simulink model "motor_speed"  (R2021b)
settings: Solver=FixedStepAuto  StartTime=0.0  StopTime=20  FixedStep=0.01  RelTol=1e-3
PreLoadFcn:
  | J = 0.01;
  | b = 0.1;
  | K = 0.01;
  | R = 1;
  | L = 0.5;
  | Ts = 0.01;
  | Kp = 210;
  | Ki = 630;
  | Kd = 20;
settings Model: Creator=adish  LastModifiedBy=adish
settings OptimizationCC: UseDivisionForNetSlopeComputation=on

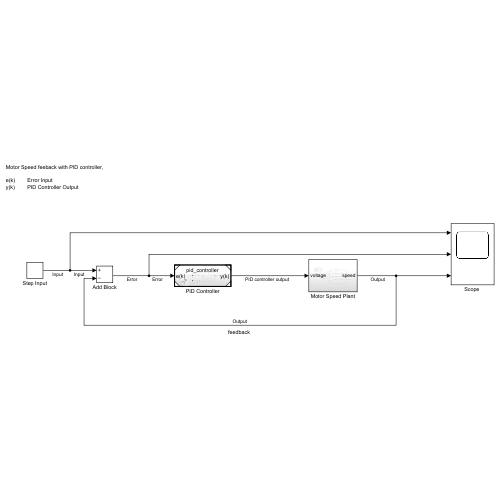
[thumbnail: Simulink's stored preview of the top-level diagram]
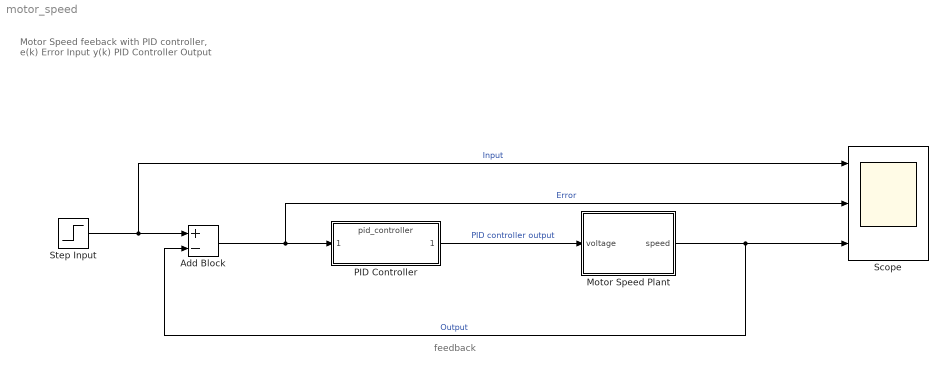
== system motor_speed ==
  note: Motor Speed feeback with PID controller,
      |
      | e(k)		Error Input
      | y(k)		PID Controller Output
  note: feedback
  Add Block : Sum  Inputs=+-
  Motor Speed Plant : Subsystem
  PID Controller : ModelReference  ModelNameDialog=pid_controller.slx  SimulationMode=Normal  ModelReferenceVersion=1.85
  "Scope " : Scope  NumInputPorts=3
  Step Input : Step  After=100  SampleTime=0
  wires:
  Step Input/1 -> "Scope "/1, Add Block/1  "Input"
  Add Block/1 -> "Scope "/2, PID Controller/1  "Error"
  PID Controller/1 -> Motor Speed Plant/1(voltage)  "PID controller output"
  Motor Speed Plant/1(speed) -> Add Block/2, "Scope "/3  "Output"

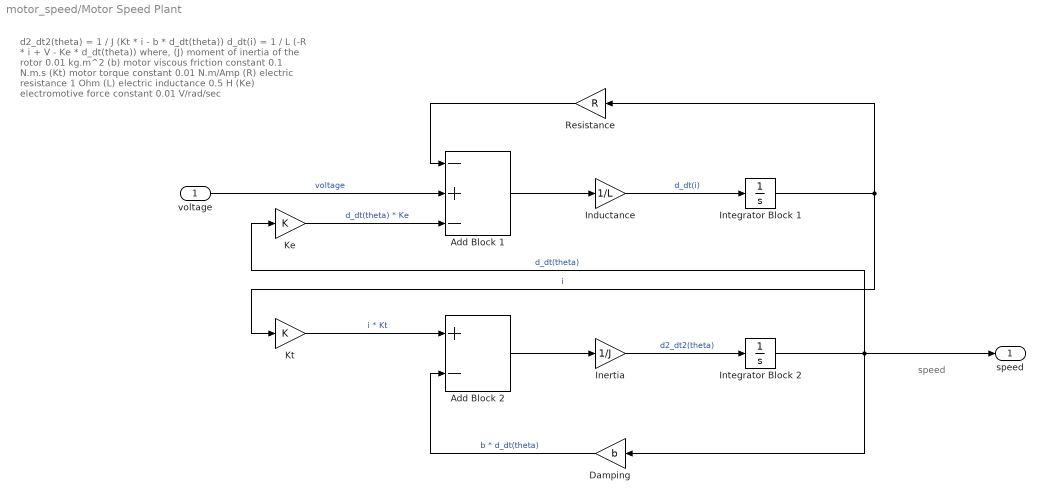
== system motor_speed/Motor Speed Plant ==
  note: speed
  note: d2_dt2(theta) = 1 / J (Kt * i - b * d_dt(theta))
      | d_dt(i) = 1 / L (-R * i + V - Ke * d_dt(theta))
      |
      | where,
      | (J) moment of inertia of the rotor 0.01 kg.m^2
      | (b) motor viscous friction constant 0.1 N.m.s
      | (Kt) motor torque constant 0.01 N.m/Amp
      | (R) electric resistance 1 Ohm
      | (L) electric inductance 0.5 H
      | (Ke) electromotive force constant 0.01 V/rad/sec
  voltage : Inport
  Add Block 1 : Sum  Inputs=-+-
  Add Block 2 : Sum  Inputs=+-
  Damping : Gain  Gain=b
  Inductance : Gain  Gain=1/L
  Inertia : Gain  Gain=1/J
  Integrator Block 1 : Integrator
  Integrator Block 2 : Integrator
  Ke : Gain  Gain=K
  Kt : Gain  Gain=K
  Resistance : Gain  Gain=R
  speed : Outport
  wires:
  Integrator Block 1/1 -> Kt/1, Resistance/1  "i"
  Add Block 2/1 -> Inertia/1
  Inertia/1 -> Integrator Block 2/1  "d2_dt2(theta)"
  Resistance/1 -> Add Block 1/1
  Add Block 1/1 -> Inductance/1
  Ke/1 -> Add Block 1/3  "d_dt(theta) * Ke"
  Damping/1 -> Add Block 2/2  "b * d_dt(theta)"
  Integrator Block 2/1 -> Damping/1, speed/1, Ke/1  "d_dt(theta)"
  Kt/1 -> Add Block 2/1  "i * Kt"
  Inductance/1 -> Integrator Block 1/1  "d_dt(i)"
  voltage/1 -> Add Block 1/2  "voltage"
